simulink model "linefollowing_array_VEX"  (R2017a)
settings: Solver=FixedStepAuto  StartTime=0.0  StopTime=inf  FixedStep=Ts  RelTol=1e-3  EnableMultiTasking=on
InitFcn:
  | Ts = 0.01;
  | axleLength = 0.28;
  | wheelR = 0.052;
  | load wheelMotorModel
  | load wheelMotorLUT
undefined symbols (not defined in the file): motorIp, motorSp
libraries: vexarmcortexlib x5, mobileRoboticsTrainingLib x1
settings Model: ExtModeTrigDuration=25  Creator=sseshadr  LastModifiedBy=shiremat
settings OptimizationCC: PassReuseOutputArgsAs=Individual arguments  MaxStackSize=64
settings DebuggingCC: ParameterTunabilityLossMsg=error
settings HardwareCC: ProdBitPerPointer=32  ProdBitPerSizeT=32  ProdBitPerPtrDiffT=32  ProdLargestAtomicInteger=Long  ProdLargestAtomicFloat=Double  ProdWordSize=32  ProdHWDeviceType=ARM Compatible->ARM Cortex
settings SFSimCC: MATLABDynamicMemAlloc=off
settings RTWCC: SystemTargetFile=ert.tlc  HardwareBoard=ARM Cortex-based VEX Microcontroller  TLCOptions="-aInlineSetEventsForThisBaseRateFcn=TLC_FALSE -aSuppressMultiTaskScheduler=TLC_FALSE  -aRateBasedStepFcn=0"  TemplateMakefile=ert_default_tmf  Description=Embedded Coder  GenerateReport=on  Toolchain=GNU Tools for VEX ARM Cortex  IncludeHyperlinkInReport=on  LaunchReport=on  GenerateTraceInfo=on  GenerateTraceReport=on  GenerateTraceReportSl=on  GenerateTraceReportSf=on  GenerateTraceReportEml=on
settings CodeAppCC: ForceParamTrailComments=on  IgnoreCustomStorageClasses=off  OperatorAnnotations=on  SimulinkDataObjDesc=on  SFDataObjDesc=on  MATLABFcnDesc=on  InsertBlockDesc=on  MATLABSourceComments=on

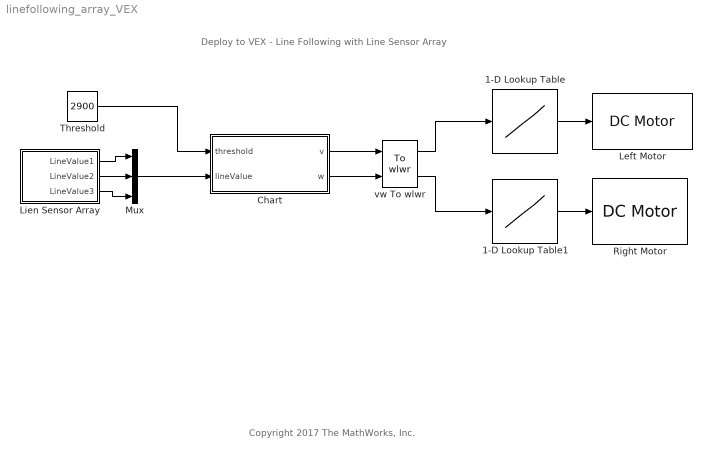
== system linefollowing_array_VEX ==
  note: Deploy to VEX - Line Following with Line Sensor Array
  note: Copyright 2017 The MathWorks, Inc.
  1-D Lookup Table : Lookup_n-D  NumberOfTableDimensions=1  BreakpointsForDimension1=motorSp  Table=motorIp  ExtrapMethod=Clip  InternalRulePriority=Speed  RndMeth=Simplest  InputSameDT=on
  1-D Lookup Table1 : Lookup_n-D  NumberOfTableDimensions=1  BreakpointsForDimension1=motorSp  Table=motorIp  ExtrapMethod=Clip  InternalRulePriority=Speed  RndMeth=Simplest  InputSameDT=on
  Chart : Stateflow chart  TreatAsAtomicUnit=on
  Left Motor : vexarmcortexlib/Actuators/DC Motor  motor=10  scaleFactor=1/13.5  SimulationOut=off
      settings: SourceProductName=Simulink Coder Support Package for ARM Cortex-based VEX Microcontroller  SourceProductBaseCode=EC_VEX_MICRO
  Lien Sensor Array : Subsystem
  Mux : Mux  Inputs=3
  Right Motor : vexarmcortexlib/Actuators/DC Motor  motor=1  scaleFactor=1/13.5  SimulationOut=off
      settings: SourceProductName=Simulink Coder Support Package for ARM Cortex-based VEX Microcontroller  SourceProductBaseCode=EC_VEX_MICRO
  Threshold : Constant  Value=2900
  vw To wlwr : mobileRoboticsTrainingLib/To wlwr  axleLength=axleLength  wheelR=wheelR
  wires:
  1-D Lookup Table1/1 -> Right Motor/1
  1-D Lookup Table/1 -> Left Motor/1
  vw To wlwr/1 -> 1-D Lookup Table/1
  vw To wlwr/2 -> 1-D Lookup Table1/1
  Chart/1(v) -> vw To wlwr/1
  Chart/2(w) -> vw To wlwr/2
  Threshold/1 -> Chart/1(threshold)
  Mux/1 -> Chart/2(lineValue)
  Lien Sensor Array/1(LineValue1) -> Mux/1
  Lien Sensor Array/2(LineValue2) -> Mux/2
  Lien Sensor Array/3(LineValue3) -> Mux/3

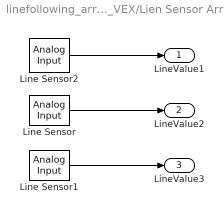
== system linefollowing_array_VEX/Lien Sensor Array ==
  Line Sensor : vexarmcortexlib/Sensors/Analog Input  inChan=7  SimulationIn=off  SampleTime=Ts
      settings: SourceProductName=Simulink Coder Support Package for ARM Cortex-based VEX Microcontroller  SourceProductBaseCode=EC_VEX_MICRO
  Line Sensor1 : vexarmcortexlib/Sensors/Analog Input  inChan=6  SimulationIn=off  SampleTime=Ts
      settings: SourceProductName=Simulink Coder Support Package for ARM Cortex-based VEX Microcontroller  SourceProductBaseCode=EC_VEX_MICRO
  Line Sensor2 : vexarmcortexlib/Sensors/Analog Input  inChan=8  SimulationIn=off  SampleTime=Ts
      settings: SourceProductName=Simulink Coder Support Package for ARM Cortex-based VEX Microcontroller  SourceProductBaseCode=EC_VEX_MICRO
  LineValue1 : Outport
  LineValue2 : Outport  Port=2
  LineValue3 : Outport  Port=3
  wires:
  Line Sensor1/1 -> LineValue3/1
  Line Sensor/1 -> LineValue2/1
  Line Sensor2/1 -> LineValue1/1

== stateflow chart linefollowing_array_VEX/Chart ==
  state FollowLine
    state Straight %StateB
      entry:
      v = 0.3;
      w = 0;
    state BearRight %StateA
      entry:
      w = -1.5;
    state BearLeft %StateC
      entry:
      w = 1.5;
    (default) -> Straight %StateB
    Straight %StateB -> BearLeft %StateC [order 1] : [lineSensor(1) < threshold]
    Straight %StateB -> BearRight %StateA [order 2] : [lineSensor(3) < threshold]
    BearRight %StateA -> Straight %StateB : [lineSensor(2) < threshold]
    BearLeft %StateC -> Straight %StateB : [lineSensor(2) < threshold]
  (default) -> FollowLine
  data: v output; w output; threshold input; lineValue input
